simulink model "InductionMachine_system_2016a"  (R2016a)
settings: Solver=VariableStepAuto  SolverMode=SingleTasking  StartTime=0.0  StopTime=10.0  RelTol=1e-3
values from neighbouring files (symbols this model uses):
  Lm = 0.01    [machinemodelvariables.m]
  Lr = Llr + Lm    (= 0.0101)    [machinemodelvariables.m]    (also in matlabderivation.m = Kr*L_abcr*Kr_inv)
  Ls = Lls + Lm    (= 0.0101)    [machinemodelvariables.m]    (also in matlabderivation.m = Ks*L_abcs*Ks_inv)
  Rr = 0.02    [machinemodelvariables.m]
  Rs = 0.12    [machinemodelvariables.m]
  Vxs = 400/(sqrt(3))    [machinemodelvariables.m]
  Vys = 0    [machinemodelvariables.m]
  wg = 2*pi*fs    (= 314.159265359)    [machinemodelvariables.m]
  wr1 = 0.98*we    (= 307.876080052)    [machinemodelvariables.m]
  wr2 = 0.97*we    (= 304.734487398)    [machinemodelvariables.m]
settings Model: Creator=Oster  LastModifiedBy=Oster
settings DataIOCC: LimitDataPoints=on  SaveOutput=off  SaveTime=off
settings OptimizationCC: BlockReduction=off  BooleanDataType=off
settings DebuggingCC: SaveWithParameterizedLinksMsg=none  UnderspecifiedInitializationDetection=Classic  MergeDetectMultiDrivingBlocksExec=none  SignalResolutionControl=TryResolveAllWithWarning  AllowSymbolicDim=off
settings HardwareCC: TargetUnknown=on
settings ConfigComp: CovMetricSettings=dwe  CovHtmlReporting=off  CovSaveCumulativeToWorkspaceVar=off  CovSaveSingleToWorkspaceVar=off  CovExternalEMLEnable=on

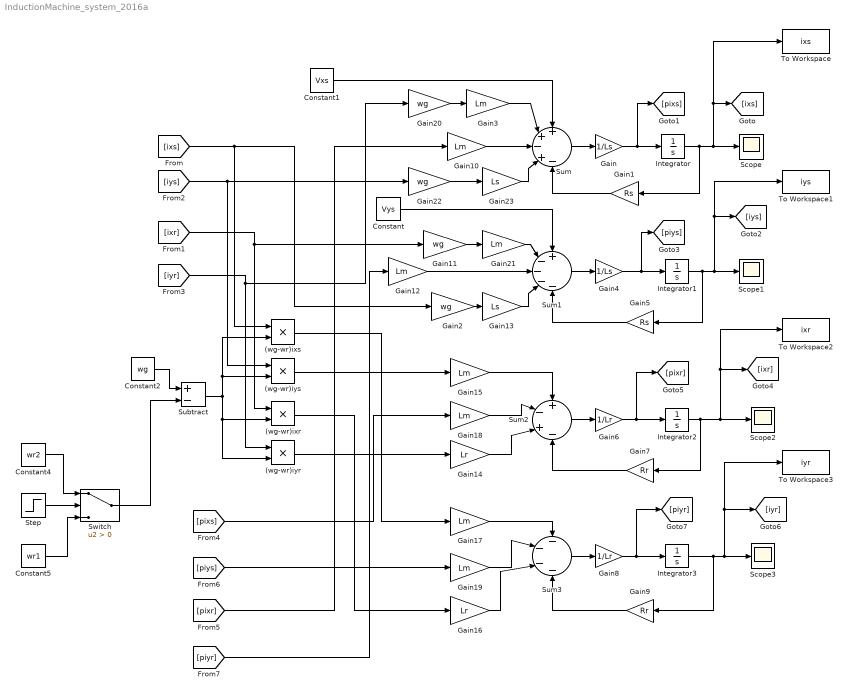
== system InductionMachine_system_2016a ==
  (wg-wr)ixr : Product
  (wg-wr)ixs : Product
  (wg-wr)iyr : Product
  (wg-wr)iys : Product
  Constant : Constant  Value=Vys
  Constant1 : Constant  Value=Vxs
  Constant2 : Constant  Value=wg
  Constant4 : Constant  Value=wr2
  Constant5 : Constant  Value=wr1
  Gain : Gain  Gain=1/Ls
  Gain1 : Gain  Gain=Rs
  Gain{3,10,12,15,17..19,21} (8 alike) : Gain  Gain=Lm
  Gain{2,11,20,22} (4 alike) : Gain  Gain=wg
  Gain13 : Gain  Gain=Ls
  Gain14 : Gain  Gain=Lr
  Gain16 : Gain  Gain=Lr
  Gain23 : Gain  Gain=Ls
  Gain4 : Gain  Gain=1/Ls
  Gain5 : Gain  Gain=Rs
  Gain6 : Gain  Gain=1/Lr
  Gain7 : Gain  Gain=Rr
  Gain8 : Gain  Gain=1/Lr
  Gain9 : Gain  Gain=Rr
  Integrator{,1..3} (4 alike) : Integrator
  Scope{,1..3} (4 alike) : Scope
  Step : Step  Before=0.97  After=0.98  SampleTime=1
  Subtract : Sum  Inputs=+-
  Sum : Sum  Inputs=++-+-
  Sum1 : Sum  Inputs=+----
  Sum2 : Sum  Inputs=+-+-
  Sum3 : Sum  Inputs=----
  Switch : Switch  Criteria=u2 > Threshold
  To Workspace : ToWorkspace  VariableName=ixs  SaveFormat=Timeseries  SampleTime=-1
  To Workspace1 : ToWorkspace  VariableName=iys  SaveFormat=Timeseries  SampleTime=-1
  To Workspace2 : ToWorkspace  VariableName=ixr  SaveFormat=Timeseries  SampleTime=-1
  To Workspace3 : ToWorkspace  VariableName=iyr  SaveFormat=Timeseries  SampleTime=-1
  wires:
  Integrator/1 -> Gain1/1, Scope/1, [ixs], To Workspace/1
  Gain/1 -> [pixs], Integrator/1
  Sum/1 -> Gain/1
  Gain1/1 -> Sum/5
  Gain3/1 -> Sum/2
  Constant1/1 -> Sum/1
  Integrator1/1 -> Gain5/1, To Workspace1/1, [iys], Scope1/1
  Gain4/1 -> [piys], Integrator1/1
  Sum1/1 -> Gain4/1
  Gain5/1 -> Sum1/5
  Integrator2/1 -> Gain7/1, To Workspace2/1, [ixr], Scope2/1
  Gain6/1 -> [pixr], Integrator2/1
  Sum2/1 -> Gain6/1
  Gain7/1 -> Sum2/4
  Integrator3/1 -> Gain9/1, To Workspace3/1, [iyr], Scope3/1
  Gain8/1 -> [piyr], Integrator3/1
  Sum3/1 -> Gain8/1
  Gain9/1 -> Sum3/4
  Constant/1 -> Sum1/1
  Gain23/1 -> Sum/4
  Gain10/1 -> Sum/3
  Gain12/1 -> Sum1/3
  Gain15/1 -> Sum2/1
  Constant2/1 -> Subtract/1
  Constant4/1 -> Switch/1
  Constant5/1 -> Switch/3
  Step/1 -> Switch/2
  Gain14/1 -> Sum2/3
  Gain16/1 -> Sum3/3
  Gain17/1 -> Sum3/1
  Subtract/1 -> (wg-wr)ixr/2, (wg-wr)iyr/2, (wg-wr)iys/2, (wg-wr)ixs/2
  [ixs] -> Gain2/1, (wg-wr)ixs/1
  [iys] -> Gain22/1, (wg-wr)iys/1
  [ixr] -> (wg-wr)ixr/1, Gain11/1
  Gain19/1 -> Sum3/2
  Gain18/1 -> Sum2/2
  [pixs] -> Gain18/1
  [piyr] -> Gain12/1
  [pixr] -> Gain10/1
  [piys] -> Gain19/1
  [iyr] -> Gain20/1, (wg-wr)iyr/1
  (wg-wr)iys/1 -> Gain15/1
  (wg-wr)ixs/1 -> Gain17/1
  (wg-wr)ixr/1 -> Gain16/1
  (wg-wr)iyr/1 -> Gain14/1
  Gain20/1 -> Gain3/1
  Gain11/1 -> Gain21/1
  Gain21/1 -> Sum1/2
  Gain22/1 -> Gain23/1
  Gain2/1 -> Gain13/1
  Gain13/1 -> Sum1/4
  Switch/1 -> Subtract/2
